simulink model "CNL_TP1_SysLinSat_SimuLink_Q22CI00_edita"  (R2018a)
settings: Solver=VariableStepAuto  StartTime=0.0  StopTime=10.0  RelTol=1e-3
settings Model: Creator=tunn  LastModifiedBy=tunn

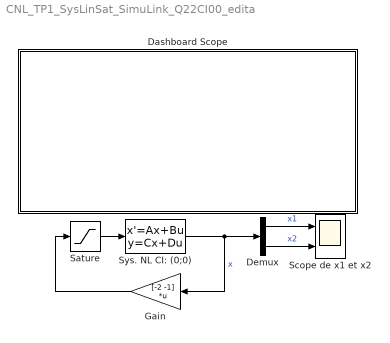
== system CNL_TP1_SysLinSat_SimuLink_Q22CI00_edita ==
  " Sys. NL CI: (0;0)" : StateSpace  A=[0 1; 1 0]  B=[0; 1]  C=eye(2)  D=[0; 0]  InitialCondition=[0; 0]
  Dashboard Scope : Subsystem  DialogController=hmiCreateDDGDialog  IsWebBlock=on  mask(MWDashboardBlock){webBlockId=6d8d5469-bd37-4983-a92c-f3284b4fdc4c, webBlockType=sdiscope, ShowInitialText=on, HMISrcModelName=CNL_TP1_SysLinSat_SimuLink_Q22CI00_edita}
      mask prompts: webBlockId "WebBlock Id"; webBlockType "WebBlock Type"; HMISrcModelName "Source Model"
      mask help: SimulinkHMI:dialogs:HMIScopeDialogDesc
      mask Help: helpview([docroot '/mapfiles/simulink.map'], 'hmi_scope')
      mask Display:
      | if strcmp(get_param(bdroot(gcb),'BlockDiagramType'), 'library')
      |     image([(matlabroot) '/toolbox/simulink/hmi/icons/DashboardScope.png']);
      | end
  Demux : Demux  Outputs=2
  Gain : Gain  Gain=[-2 -1]  Multiplication=Matrix(K*u)
  Sature : Saturate  UpperLimit=1  LowerLimit=-1
  Scope de x1 et x2 : Scope  NumInputPorts=2
  wires:
  " Sys. NL CI: (0;0)"/1 -> Gain/1, Demux/1  "x"
  Demux/2 -> Scope de x1 et x2/2  "x2"
  Demux/1 -> Scope de x1 et x2/1  "x1"
  Sature/1 -> " Sys. NL CI: (0;0)"/1
  Gain/1 -> Sature/1

== system CNL_TP1_SysLinSat_SimuLink_Q22CI00_edita/Dashboard Scope ==
